simulink model "si4_forced_oscillator"  (R2024a)
settings: Solver=VariableStepAuto  StartTime=0.0  StopTime=te  RelTol=1e-3  EnableMultiTasking=on
values from neighbouring files (symbols this model uses):
  c = -0.8    [si5_Ball_parameter.m]    (also in sim21_ODE.m = 1)
  F = 1    [sim21_ODE.m]
  k = 10    [si5_Ball_parameter.m]    (also in sim21_ODE.m = 3)
  m = 0.35    [Electromagnet_par.m]    (also in si5_Ball_parameter.m = 0.1; sim21_ODE.m = 3)
  w = 2*pi/0.1    (= 62.8318530718)    [Electromagnet_par.m]    (also in coil_ironcore.m = 314.159265359; sim21_ODE.m = [0.5 1 2])
  x0 = 0.01    [Electromagnet_par.m]    (also in sim21_ODE.m = [0 0])
settings Model: Creator=sar  LastModifiedBy=ocean
settings SolverCC: AlgebraicLoopSolver=TrustRegion
settings DataIOCC: LimitDataPoints=on  ReturnWorkspaceOutputs=off  Refine=10
settings OptimizationCC: LifeSpan=inf
settings DebuggingCC: UnconnectedInputMsg=warning  UnconnectedOutputMsg=warning  UnconnectedLineMsg=warning  AllowSymbolicDim=off  SFUnexpectedBacktrackingDiag=warning  SFNoUnconditionalDefaultTransitionDiag=warning  SFExecutionAtInitializationDiag=none  ArithmeticOperatorsInVariantConditions=warning
settings ModelReferenceCC: EnableRefExpFcnMdlSchedulingChecks=on  PropagateSignalLabelsOutOfModel=off
settings SFSimCC: SimUseLocalCustomCode=off  CustomCodeUndefinedFunction=UseInterfaceOnly
settings RTWCC: RTWUseLocalCustomCode=off  GPUComputeCapability=3.5  DLArmComputeVersion=19.05
settings CodeAppCC: StateflowObjectComments=on
settings GRTTargetCC: TargetLangStandard=C89/C90 (ANSI)
settings ConfigComp: CovMetricSettings=dw  CovSaveCumulativeToWorkspaceVar=on  CovSaveSingleToWorkspaceVar=on  CovExternalEMLEnable=off

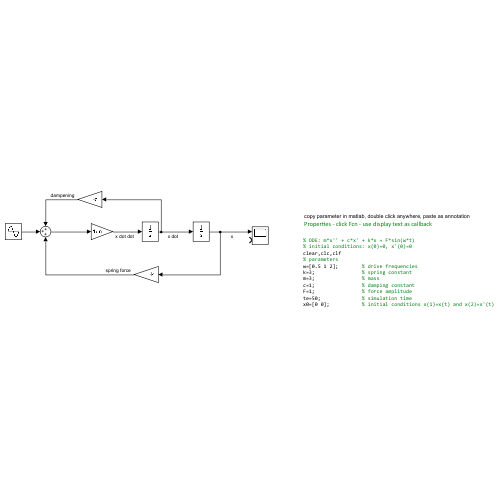
[thumbnail: Simulink's stored preview of the top-level diagram]
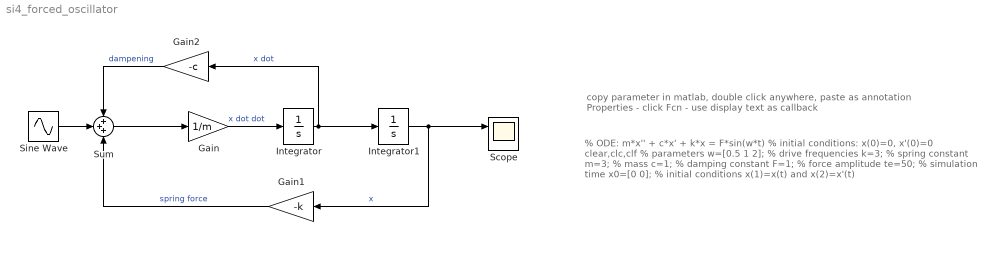
== system si4_forced_oscillator ==
  note: copy parameter in matlab, double click anywhere, paste as annotation
      | Properties - click Fcn - use display text as callback
  note: % ODE: m*x'' + c*x' + k*x = F*sin(w*t)
      | % initial conditions: x(0)=0, x'(0)=0
      | clear,clc,clf
      | % parameters
      | w=[0.5 1 2]; % drive frequencies
      | k=3; % spring constant
      | m=3; % mass
      | c=1; % damping constant
      | F=1; % force amplitude
      | te=50; % simulation time
      | x0=[0 0]; % initial conditions x(1)=x(t) and x(2)=x'(t)
  Gain : Gain  Gain=1/m
  Gain1 : Gain  Gain=-k
  Gain2 : Gain  Gain=-c
  Integrator : Integrator  InitialCondition=x0(2)
  Integrator1 : Integrator  InitialCondition=x0(1)
  Scope : Scope  NumInputPorts=2
  Sine Wave : Sin  Amplitude=F  Frequency=w  SampleTime=0
  Sum : Sum  Inputs=+++
  wires:
  Gain/1 -> Integrator/1  "x dot dot"
  Integrator/1 -> Gain2/1, Integrator1/1  "x dot"
  Integrator1/1 -> Gain1/1, Scope/1  "x"
  Gain2/1 -> Sum/1  "dampening"
  Sum/1 -> Gain/1
  Sine Wave/1 -> Sum/2
  Gain1/1 -> Sum/3  "spring force"
